simulink model "sim2"  (R2024a)
settings: Solver=FixedStepAuto  StartTime=0.0  StopTime=70.0  FixedStep=1  RelTol=1e-3
settings Model: Creator=alexe  LastModifiedBy=alexe

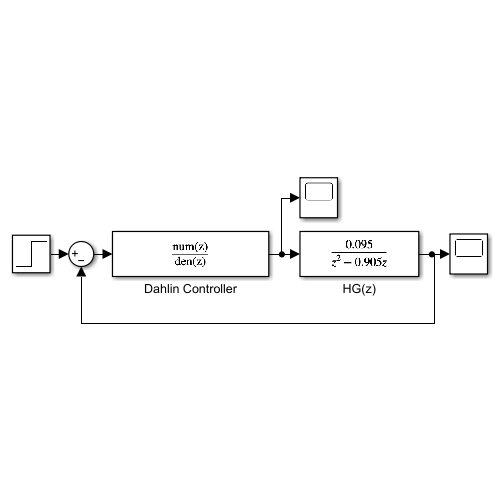
[thumbnail: Simulink's stored preview of the top-level diagram]
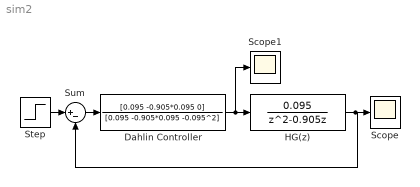
== system sim2 ==
  Dahlin Controller : DiscreteTransferFcn  Numerator=[0.095 -0.905*0.095 0]  Denominator=[0.095 -0.905*0.095 -0.095^2]
  HG(z) : DiscreteTransferFcn  Numerator=[0 0 0.095]  Denominator=[1 -0.905 0]
  Scope : Scope
  Scope1 : Scope
  Step : Step  Before=1
  Sum : Sum  Inputs=|+-
  wires:
  Step/1 -> Sum/1
  Sum/1 -> Dahlin Controller/1
  Dahlin Controller/1 -> Scope1/1, HG(z)/1
  HG(z)/1 -> Sum/2, Scope/1
